simulink model "Longi_Param_Recog"  (R2023a)
settings: Solver=VariableStepAuto  StartTime=0.0  StopTime=40  RelTol=1e-3
libraries: simulink x3
settings Model: Creator=28303  LastModifiedBy=28303

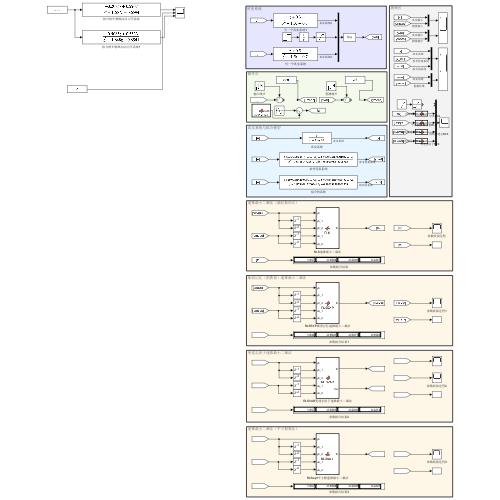
[thumbnail: Simulink's stored preview of the top-level diagram]
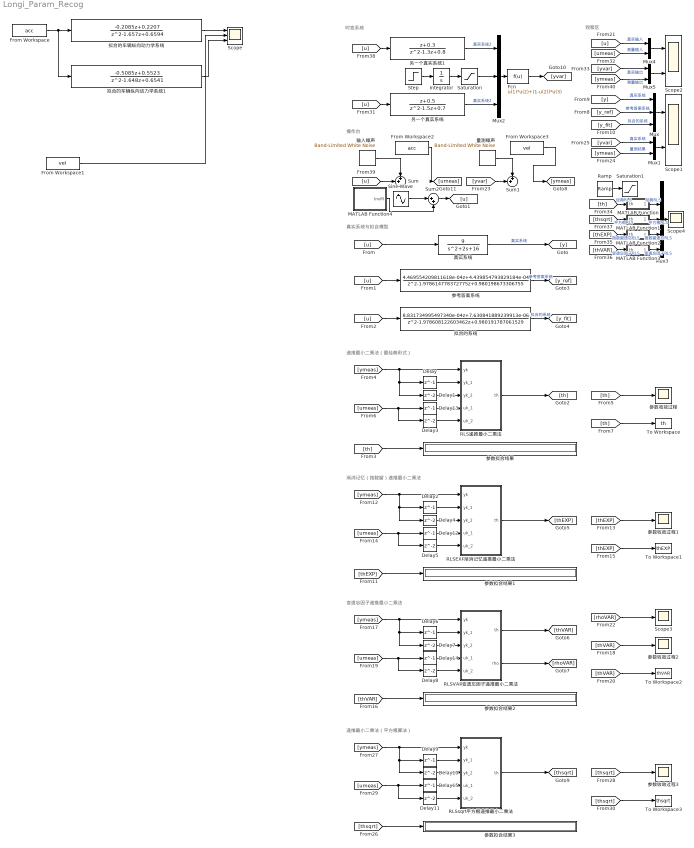
== system Longi_Param_Recog ==
  note: 时变系统
  note: 观察区
  note: 真实系统与拟合模型
  note: 渐消记忆（指数窗）递推最小二乘法
  note: 递推最小二乘法（最经典形式）
  note: 递推最小二乘法（平方根算法）
  note: 变遗忘因子递推最小二乘法
  note: 操作台
  Delay{,2,6,9,12..15} (8 alike) : Delay  DelayLength=1  SampleTime=0.01
  Delay{1,3..5,7..8,10..11} (8 alike) : Delay  SampleTime=0.01
  Fcn : Fcn  Expr=u(1)*u(2)+(1-u(2))*u(3)
  From Workspace : FromWorkspace  VariableName=acc
  From Workspace1 : FromWorkspace  VariableName=vel
  From Workspace2 : FromWorkspace  VariableName=acc
  From Workspace3 : FromWorkspace  VariableName=vel
  Integrator : Integrator
  MATLAB Function : MATLAB Function  TreatAsAtomicUnit=on
  MATLAB Function1 : MATLAB Function  TreatAsAtomicUnit=on
  MATLAB Function2 : MATLAB Function  TreatAsAtomicUnit=on
  MATLAB Function3 : MATLAB Function  TreatAsAtomicUnit=on
  MATLAB Function4 : MATLAB Function  TreatAsAtomicUnit=on  SystemSampleTime=0.05
  Mux : Mux  Inputs=3
  Mux1 : Mux  Inputs=2
  Mux2 : Mux  Inputs=3
  Mux3 : Mux  Inputs=5
  Mux4 : Mux  Inputs=2
  Mux5 : Mux  Inputs=2
  "RLSEXP渐消记忆递推最小二乘法 " : MATLAB Function  TreatAsAtomicUnit=on  SystemSampleTime=0.01
  "RLSVAR变遗忘因子递推最小二乘法 " : MATLAB Function  TreatAsAtomicUnit=on  SystemSampleTime=0.01
  "RLSsqrt平方根递推最小二乘法 " : MATLAB Function  TreatAsAtomicUnit=on  SystemSampleTime=0.01
  "RLS递推最小二乘法 " : MATLAB Function  TreatAsAtomicUnit=on  SystemSampleTime=0.01
  Ramp : simulink/Sources/Ramp  slope=-0.5  start=4.5  InitialOutput=2.3
  Saturation : Saturate  UpperLimit=1  LowerLimit=0
  Saturation1 : Saturate  UpperLimit=5  LowerLimit=1.8
  Scope : Scope  NumInputPorts=3
  Scope1 : Scope  NumInputPorts=2
  Scope2 : Scope  NumInputPorts=2
  Scope3 : Scope
  Scope4 : Scope
  Sine Wave : Sin  Amplitude=2  SampleTime=0
  Step : Step  Time=4.5  SampleTime=0
  Sum : Sum  Inputs=++|
  Sum1 : Sum  Inputs=++|
  Sum2 : Sum  Inputs=|++
  To Workspace : ToWorkspace  VariableName=th  SaveFormat=Timeseries  SampleTime=-1
  To Workspace1 : ToWorkspace  VariableName=thEXP  SaveFormat=Timeseries  SampleTime=-1
  To Workspace2 : ToWorkspace  VariableName=thVAR  SaveFormat=Timeseries  SampleTime=-1
  To Workspace3 : ToWorkspace  VariableName=thsqrt  SaveFormat=Timeseries  SampleTime=-1
  参数拟合结果{,1..3} (4 alike) : Display
  参数收敛过程{,1..3} (4 alike) : Scope
  参考答案系统 : DiscreteTransferFcn  Numerator=[4.469554209811618e-04 4.439854793829184e-04]  Denominator=[1 -1.978614778372775 0.980198673306755]
  另一个真实系统 : DiscreteTransferFcn  Numerator=[0 1 0.5]  Denominator=[1 -1.5 0.7]
  另一个真实系统1 : DiscreteTransferFcn  Numerator=[0 1 0.3]  Denominator=[1 -1.3 0.8]
  拟合的系统 : DiscreteTransferFcn  Numerator=[8.831734995497340e-04 7.630841889239913e-06]  Denominator=[1 -1.978608122603462 0.980191787061529]
  拟合的车辆纵向动力学系统 : DiscreteTransferFcn  Numerator=[-0.2085 0.2207]  Denominator=[1 -1.657 0.6594]
  拟合的车辆纵向动力学系统1 : DiscreteTransferFcn  Numerator=[-0.5085 0.5523]  Denominator=[1 -1.648 0.6541]
  真实系统 : TransferFcn  Numerator=[9]  Denominator=[1 2 16]
  输入噪声 : simulink/Sources/Band-Limited White Noise  Cov=0.01  Ts=0.1  seed=[32141]
  量测噪声 : simulink/Sources/Band-Limited White Noise  Cov=0.01  Ts=0.01  seed=[233341]
  wires:
  From Workspace/1 -> 拟合的车辆纵向动力学系统1/1, 拟合的车辆纵向动力学系统/1
  拟合的车辆纵向动力学系统/1 -> Scope/1
  From Workspace1/1 -> Scope/2
  Delay9/1 -> "RLSsqrt平方根递推最小二乘法 "/2(yk_1)
  MATLAB Function4/1(InvM) -> Sum2/2
  Saturation/1 -> Mux2/2
  Mux2/1 -> Fcn/1
  Sum2/1 -> [u]
  [yvar] -> Mux1/1  "真实系统"
  [ymeas] -> "RLSEXP渐消记忆递推最小二乘法 "/1(yk), Delay2/1, Delay4/1
  另一个真实系统/1 -> Mux2/3  "真实系统2"
  Delay3/1 -> "RLS递推最小二乘法 "/5(uk_2)
  Mux5/1 -> Scope2/2
  Mux4/1 -> Scope2/1
  Sine Wave/1 -> Sum2/1
  Fcn/1 -> [yvar]
  Delay15/1 -> "RLSsqrt平方根递推最小二乘法 "/4(uk_1)
  Delay2/1 -> "RLSEXP渐消记忆递推最小二乘法 "/2(yk_1)
  [umeas] -> Mux4/2  "测量输入"
  Integrator/1 -> Saturation/1
  [thVAR] -> 参数收敛过程2/1
  MATLAB Function3/1(output) -> Mux3/5  "变遗忘因子RLS"
  Ramp/1 -> Saturation1/1
  Delay8/1 -> "RLSVAR变遗忘因子递推最小二乘法 "/5(uk_2)
  MATLAB Function/1(output) -> Mux3/2  "经典RLS"
  MATLAB Function2/1(output) -> Mux3/4  "指数窗遗忘RLS"
  [y_ref] -> Mux/2  "参考答案系统"
  [yvar] -> Mux5/1  "真实输出"
  [u] -> Mux4/1  "真实输入"
  Mux3/1 -> Scope4/1
  Delay6/1 -> "RLSVAR变遗忘因子递推最小二乘法 "/2(yk_1)
  [ymeas] -> Delay1/1, Delay/1, "RLS递推最小二乘法 "/1(yk)
  Delay13/1 -> "RLS递推最小二乘法 "/4(uk_1)
  Mux/1 -> Scope1/1
  Step/1 -> Integrator/1
  Delay10/1 -> "RLSsqrt平方根递推最小二乘法 "/3(yk_2)
  另一个真实系统1/1 -> Mux2/1  "真实系统2"
  Delay11/1 -> "RLSsqrt平方根递推最小二乘法 "/5(uk_2)
  [thEXP] -> MATLAB Function2/1(th)  "指数窗遗忘RLS"
  [u] -> Sum/2
  [u] -> 另一个真实系统1/1
  [thsqrt] -> MATLAB Function1/1(th)  "平方根RLS"
  输入噪声/1 -> Sum/1
  Delay12/1 -> "RLSEXP渐消记忆递推最小二乘法 "/4(uk_1)
  [umeas] -> Delay3/1, Delay13/1
  [umeas] -> Delay15/1, Delay11/1
  "RLSsqrt平方根递推最小二乘法 "/1(th) -> [thsqrt]
  [thsqrt] -> 参数拟合结果3/1
  [umeas] -> Delay12/1, Delay5/1
  [ymeas] -> "RLSsqrt平方根递推最小二乘法 "/1(yk), Delay9/1, Delay10/1
  MATLAB Function1/1(output) -> Mux3/3  "平方根RLS"
  [thEXP] -> To Workspace1/1
  [thEXP] -> 参数拟合结果1/1
  [y_fit] -> Mux/3  "拟合的系统"
  量测噪声/1 -> Sum1/1
  "RLSVAR变遗忘因子递推最小二乘法 "/1(th) -> [thVAR]
  [thVAR] -> To Workspace2/1
  [th] -> MATLAB Function/1(th)  "经典RLS"
  [yvar] -> Sum1/2
  [u] -> 另一个真实系统/1
  [rhoVAR] -> Scope3/1
  [ymeas] -> Delay7/1, Delay6/1, "RLSVAR变遗忘因子递推最小二乘法 "/1(yk)
  [umeas] -> Delay14/1, Delay8/1
  [ymeas] -> Mux1/2  "量测结果"
  [thVAR] -> 参数拟合结果2/1
  [thsqrt] -> To Workspace3/1
  "RLSVAR变遗忘因子递推最小二乘法 "/2(rho) -> [rhoVAR]
  [thsqrt] -> 参数收敛过程3/1
  [y] -> Mux/1  "真实系统"
  [thVAR] -> MATLAB Function3/1(th)  "变遗忘因子RLS"
  [thEXP] -> 参数收敛过程1/1
  Delay4/1 -> "RLSEXP渐消记忆递推最小二乘法 "/3(yk_2)
  Mux1/1 -> Scope1/2
  [th] -> 参数收敛过程/1
  拟合的系统/1 -> [y_fit]  "拟合的系统"
  [ymeas] -> Mux5/2  "测量输出"
  参考答案系统/1 -> [y_ref]  "参考答案系统"
  [u] -> 参考答案系统/1
  Delay5/1 -> "RLSEXP渐消记忆递推最小二乘法 "/5(uk_2)
  [th] -> To Workspace/1
  [th] -> 参数拟合结果/1
  "RLSEXP渐消记忆递推最小二乘法 "/1(th) -> [thEXP]
  Delay14/1 -> "RLSVAR变遗忘因子递推最小二乘法 "/4(uk_1)
  Delay7/1 -> "RLSVAR变遗忘因子递推最小二乘法 "/3(yk_2)
  [u] -> 真实系统/1
  "RLS递推最小二乘法 "/1(th) -> [th]
  Delay/1 -> "RLS递推最小二乘法 "/2(yk_1)
  真实系统/1 -> [y]  "真实系统"
  Delay1/1 -> "RLS递推最小二乘法 "/3(yk_2)
  [u] -> 拟合的系统/1
  From Workspace2/1 -> [umeas]
  From Workspace3/1 -> [ymeas]
  拟合的车辆纵向动力学系统1/1 -> Scope/3

== matlab function Longi_Param_Recog/RLSEXP渐消记忆递推最小二乘法  ==
  data: yk input; th output; yk_1 input; yk_2 input; uk_1 input; uk_2 input
function th = RLSEXP(yk,yk_1,yk_2,uk_1,uk_2)
%选取遗忘因子的准则：rho=1-1/N,N为想要记忆的历史数据长度
%比如N=100，则rho=0.99；
persistent th0 P0 rho
if isempty(th0)
    th0=zeros(4,1);
    P0=eye(4)*2e3;
    rho=0.99;
end
fai=[yk_1,yk_2,uk_1,uk_2]';

th=th0+P0*fai/(fai'*P0*fai+rho)*(yk-fai'*th0);
P0=(P0-P0*(fai*fai')*P0/(fai'*P0*fai+1))/rho;
th0=th;

end

== matlab function Longi_Param_Recog/RLS递推最小二乘法  ==
  data: yk input; th output; yk_1 input; yk_2 input; uk_1 input; uk_2 input
function th = RLS(yk,yk_1,yk_2,uk_1,uk_2)
persistent th0 P0
if isempty(th0)
    th0=zeros(4,1);
    P0=eye(4)*2e3;
end
fai=[yk_1,yk_2,uk_1,uk_2]';

th=th0+P0*fai/(fai'*P0*fai+1)*(yk-fai'*th0);
P0=P0-P0*(fai*fai')*P0/(fai'*P0*fai+1);
th0=th;

end

== matlab function Longi_Param_Recog/RLSVAR变遗忘因子递推最小二乘法  ==
  data: yk input; th output; yk_1 input; yk_2 input; uk_1 input; uk_2 input; rho output
function [th,rho] = RLSVAR(yk,yk_1,yk_2,uk_1,uk_2)

persistent th0 P0 Sigma rhomin
if isempty(th0)
    th0=zeros(4,1);
    P0=eye(4)*2e3;
    N=500;      %一般记忆步长
    Nmin=50;    %最小记忆步长
    sig02=0.02; %观察噪声方差
    Sigma=sig02*N;
    rhomin=1-1/Nmin;
end
fai=[yk_1,yk_2,uk_1,uk_2]';
ek=(yk-fai'*th0);           %计算本步预测误差
K=P0*fai/(fai'*P0*fai+1);   %计算增益
th=th0+K*ek;                %修正估计
rho=1-(1-fai'*K)*ek^2/Sigma;%计算遗忘因子
if rho<rhomin               %防止遗忘因子过小
    rho=rhomin;
end
P0=(P0-P0*(fai*fai')*P0/(fai'*P0*fai+1))/rho;%更新协方差
th0=th;%更新记忆数据

end

== matlab function Longi_Param_Recog/RLSsqrt平方根递推最小二乘法  ==
  data: yk input; th output; yk_1 input; yk_2 input; uk_1 input; uk_2 input
function th = RLSsqrt(yk,yk_1,yk_2,uk_1,uk_2)
persistent th0 S0
if isempty(th0)
    th0=zeros(4,1);
    S0=eye(4)*sqrt(2e3);
end
fai=[yk_1,yk_2,uk_1,uk_2]';%构造向量fai
f=S0'*fai;
g=1/(f'*f+1);
a=1/(1+sqrt(g));
K=S0*f*g;
th=th0+K*(yk-fai'*th0);
S0=S0*(eye(4)-g*a*(f*f'));
th0=th;

end

== matlab function Longi_Param_Recog/MATLAB Function ==
  data: th input; output output
function output = fcn(th)
output=sum(th);
end

== matlab function Longi_Param_Recog/MATLAB Function1 ==
  data: th input; output output
function output = fcn(th)
output=sum(th);
end

== matlab function Longi_Param_Recog/MATLAB Function2 ==
  data: th input; output output
function output = fcn(th)
output=sum(th);
end

== matlab function Longi_Param_Recog/MATLAB Function3 ==
  data: th input; output output
function output = fcn(th)
output=sum(th);
end

== matlab function Longi_Param_Recog/MATLAB Function4 ==
  data: InvM output
function InvM = InvMseries()
coder.extrinsic('idinput')
persistent ms i S gain
if isempty(ms)
   i=1;
   n=15;
   p=2^n-1;
   S=false;
   ms=zeros(p,1);
   ms0=idinput(p,'prbs',[],[0 1]);
   ms(1:end,1)=ms0(1:p,1);
   gain=5;
end
flag=true;
if ms(i)==0
    flag=false;
end
invm=xor(S,flag);
if invm
    InvM=gain;
else
    InvM=-gain;
end

i=i+1;
S=not(S);


end
